simulink model "PRGCRCDEMO"  (R2014b)
settings: Solver=FixedStepDiscrete  StartTime=0.0  StopTime=10.0  FixedStep=1e-3  RelTol=1e-3
PreLoadFcn:
  | Hyo_customization
undefined symbols (not defined in the file): _EngStat, _Init, _Read_len32, _Write_32_bit, chklen, CRC, crcseed, encrcint, endma, eninbits, eninbytes, enoutbits, enoutbytes, indatasize, noparam, polyval, s6j3200_PRGCRC, xordata
libraries: periblklib x5
settings Model: Creator=Hyowinner  LastModifiedBy=Hyowinner
settings OptimizationCC: InlineParams=on  OptimizeModelRefInitCode=on  LifeSpan=1
settings HardwareCC: ProdLargestAtomicInteger=Integer  ProdLargestAtomicFloat=Float  ProdIntDivRoundTo=Zero  ProdEndianess=LittleEndian  ProdHWDeviceType=CYPRESS->ARM Cortex-R5
settings RTWCC: SystemTargetFile=Hyo.tlc  GenCodeOnly=on  MakeCommand=none  GenerateMakefile=off  TemplateMakefile=none  Description=System Target File for S6J3200 Series MCU Target  GenerateReport=on  ProcessScript=Hyo_make_rtw_hook  IncludeHyperlinkInReport=on  LaunchReport=on
settings CodeAppCC: IgnoreCustomStorageClasses=off
settings STFCustomTargetCC: ModelReferenceCompliant=off  IncludeMdlTerminateFcn=off  CombineOutputUpdateFcns=on  ERTFirstTimeCompliant=on  ERTCustomFileBanners=on  SupportContinuousTime=off  SupportNonInlinedSFcns=off  MATLABClassNameForMDSCustomization=Simulink.SoftwareTarget.ERTCustomization  GRTInterface=off  SystemTargetFile=Hyo.tlc
settings ERTTargetCC: ModelReferenceCompliant=off  ParMdlRefBuildCompliant=off  CompOptLevelCompliant=off  ConcurrentExecutionCompliant=off  IncludeMdlTerminateFcn=off  ModelStepFunctionPrototypeControlCompliant=off  CPPClassGenCompliant=off  InlinedParameterPlacement=NonHierarchical  ERTSrcFileBannerTemplate=Hyo_code_template.cgt  ERTHdrFileBannerTemplate=Hyo_code_template.cgt  ERTDataSrcFileTemplate=Hyo_code_template.cgt  ERTDataHdrFileTemplate=Hyo_code_template.cgt  ERTCustomFileTemplate=example_file_process.tlc  EnableUserReplacementTypes=on

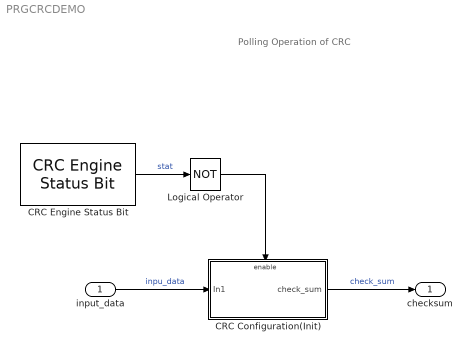
== system PRGCRCDEMO ==
  note: Polling Operation of CRC
  input_data : Inport  OutDataTypeStr=uint_io32_t
  CRC Configuration(Init) : Subsystem  TreatAsAtomicUnit=on
  CRC Engine Status Bit : periblklib/Programmable CRC/CRC Engine Status Bit  g_pv=s6j3200_PRGCRC.h,CRC,_EngStat;noparam,noparam;
  Logical Operator : Logic  Operator=NOT  Inputs=1  AllPortsSameDT=off  OutDataTypeStr=boolean
  checksum : Outport
  wires:
  CRC Engine Status Bit/1 -> Logical Operator/1  "stat"
  Logical Operator/1 -> CRC Configuration(Init)/Enable
  input_data/1 -> CRC Configuration(Init)/1(In1)  "inpu_data"
  CRC Configuration(Init)/1(check_sum) -> checksum/1  "check_sum"

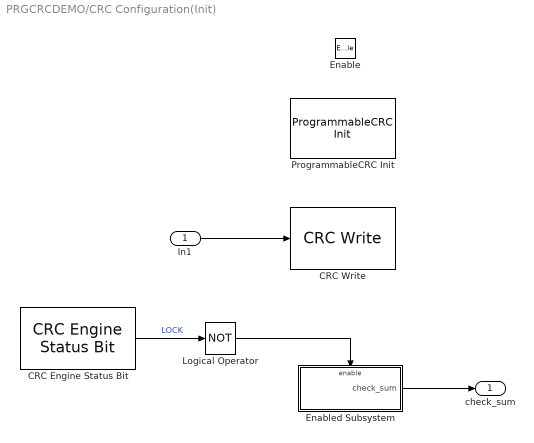
== system PRGCRCDEMO/CRC Configuration(Init) ==
  In1 : Inport
  Enable : EnablePort
  CRC Engine Status Bit : periblklib/Programmable CRC/CRC Engine Status Bit  g_pv=s6j3200_PRGCRC.h,CRC,_EngStat;noparam,noparam;
  CRC Write : periblklib/Programmable CRC/CRC Write  Priority=-1  g_pv=s6j3200_PRGCRC.h,CRC,_Write_32_bit;indatasize,32_bit;
  Enabled Subsystem : Subsystem  TreatAsAtomicUnit=on
  Logical Operator : Logic  Operator=NOT  AllPortsSameDT=off  OutDataTypeStr=boolean
  ProgrammableCRC Init : periblklib/Programmable CRC/ProgrammableCRC Init  g_pv=s6j3200_PRGCRC.h,CRC,_Init;polyval,0x04C11DB7;crcseed,0xFFFFFFFF;xordata,0xFFFFFFFF;endma,on;encrcint,off;indatasize,32_bit;chklen,32;eninbits,off;eninbytes,off;enoutbits,off;enoutbytes,off;
  check_sum : Outport  OutDataTypeStr=uint_io32_t
  wires:
  In1/1 -> CRC Write/1
  CRC Engine Status Bit/1 -> Logical Operator/1  "LOCK"
  Enabled Subsystem/1(check_sum) -> check_sum/1
  Logical Operator/1 -> Enabled Subsystem/Enable

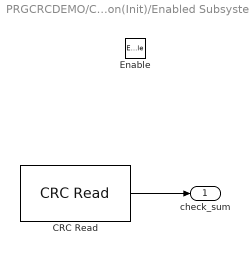
== system PRGCRCDEMO/CRC Configuration(Init)/Enabled Subsystem ==
  Enable : EnablePort
  CRC Read : periblklib/Programmable CRC/CRC Read  g_pv=s6j3200_PRGCRC.h,CRC,_Read_len32;chklen,32;
  check_sum : Outport  OutDataTypeStr=uint_io32_t
  wires:
  CRC Read/1 -> check_sum/1
